simulink model "vehicle_model_paper_2017"  (R2019b)
settings: Solver=ode15s  StartTime=0.0  StopTime=30  RelTol=1e-3  AbsTol=1e-6
values from neighbouring files (symbols this model uses):
  Cr = 0.015    [parameter_values.m]
  Ctr_data = [2.2320 2.0750 1.9750 1.8460 1.7200 1.5640 1.4090 1.2540 1.0960 1.0800 1.0610 1.0430 1.0280 1.0120 1.002 1.002 1.001 0.9980 0.9990 1.001 1.002]    [parameter_values.m]
  DOWN_TABLE = [ ... (first row only)    [parameter_values.m]
  DOWN_TH_BP = [0 2.2352 17.8816 22.352 40.2336 44.704]    [parameter_values.m]
  g = 9.8    [parameter_values.m]
  gear_ratio = [2.34 1.450 1.000 0.68]    [parameter_values.m]
  Iei = 0.224    [parameter_values.m]
  Kb = 20    [parameter_values.m]
  Kc = 1    [parameter_values.m]
  Ktc_data = [ 137.4652 137.0650 135.8644 135.6644 137.5653 140.3666 145.2689 152.8725 162.9773 164.2779 166.1788 167.9797 170.0807 172.7820 175.3832 179.5852 183.5871 189.8901  197.6938 215.9024 244.5160 ]    [parameter_values.m]
  Ktc_ni_ne = [0 0.1000 0.2000 0.3000 0.4000 0.5000 0.6000 0.7000 0.8000 0.8100 0.8200 0.8300 0.8400 0.8500 0.8600 0.8700 0.8800 0.8900 0.9000 0.9200 0.9400]    [parameter_values.m]
  m = 1500.5    [parameter_values.m]
  r = 0.326    [parameter_values.m]
  Rf = 3.28    [parameter_values.m]
  rhoACd = 0.98    [parameter_values.m]
  taub = 0.2    [parameter_values.m]
  Te_data = [ ... (first row only)    [parameter_values.m]
  Te_rpm = [800:400:4800]    [parameter_values.m]
  Te_throtle = [0 20 30 40 50 60 70 80 90 100] / 100    [parameter_values.m]
  UP_TABLE = [ ... (first row only)    [parameter_values.m]
  UP_TH_BP = [ 0 11.176 15.6464 22.352 40.2336 44.704]    [parameter_values.m]
undefined symbols (not defined in the file or in its folder): sigbuilder_block
settings Model: DataTypeOverride=Double  MinMaxOverflowLogging=ForceOff  Creator=ignisgravitas  LastModifiedBy=sls-1
settings SolverCC: MaxOrder=2
settings DebuggingCC: ArithmeticOperatorsInVariantConditions=warning
settings SFSimCC: CustomCodeUndefinedFunction=UseInterfaceOnly

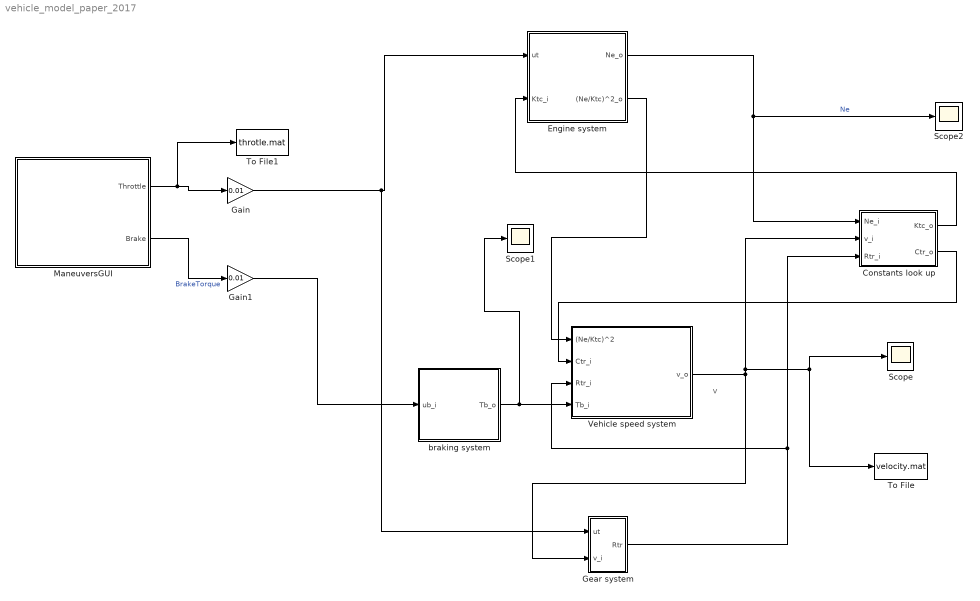
== system vehicle_model_paper_2017 ==
  note: v
  Constants look up : Subsystem
  Engine system : Subsystem
  Gain : Gain  Gain=0.01
  Gain1 : Gain  Gain=0.01
  Gear system : Subsystem
  ManeuversGUI : Subsystem  Tag=STV Subsys  LoadFcn=sigbuilder_block('load');  StartFcn=sigbuilder_block('start');  StopFcn=sigbuilder_block('stop');  ClipboardFcn=sigbuilder_block('clipboard');  mask(Sigbuilder block){tuvar=[0:10]}
      mask help: Sigbuilder GUI
      mask init:
      | tuvar = sigbuilder_block('maskInit');
      settings: CopyFcn=sigbuilder_block('copy');  DeleteFcn=sigbuilder_block('delete');  ModelCloseFcn=sigbuilder_block('modelClose');  PreSaveFcn=sigbuilder_block('preSave');  PauseFcn=sigbuilder_block('pause')  ContinueFcn=sigbuilder_block('continue')  NameChangeFcn=sigbuilder_block('namechange');  OpenFcn=sigbuilder_block('open',[152.337 144.758 981.474 499.453 ]);  CloseFcn=sigbuilder_block('close');
      mask Display: plot(0, 0, 100, 100,[2, 2, 32, 32, 2], [68, 8, 8, 68, 68],[32, 2], [38, 38], [32, 19, 2],[53, 60, 44], [32, 17, 17, 2],[16, 16, 31, 31]);txt = getActiveGroup(gcbh);text(2, 100, txt,'verticalAlignment', 'top');
  Scope : Scope
  Scope1 : Scope
  Scope2 : Scope
  To File : ToFile  Filename=velocity.mat  MatrixName=velocity  SaveFormat=Timeseries
  To File1 : ToFile  Filename=throtle.mat  MatrixName=throtle  SaveFormat=Timeseries
  Vehicle speed system : Subsystem
  braking system : Subsystem
  wires:
  Vehicle speed system/1(v_o) -> To File/1, Scope/1, Constants look up/2(v_i), Gear system/2(v_i)
  Constants look up/2("Ctr_o ") -> Vehicle speed system/2(Ctr_i)
  braking system/1(Tb_o) -> Scope1/1, Vehicle speed system/4(Tb_i)
  Engine system/1(Ne_o) -> Scope2/1, Constants look up/1(Ne_i)  "Ne"
  Engine system/2((Ne/Ktc)^2_o) -> Vehicle speed system/1((Ne/Ktc)^2)
  Gear system/1(Rtr) -> Constants look up/3(Rtr_i), Vehicle speed system/3(Rtr_i)
  ManeuversGUI/1(Throttle) -> To File1/1, Gain/1
  Gain/1 -> Gear system/1(ut), Engine system/1(ut)
  ManeuversGUI/2(Brake) -> Gain1/1  "BrakeTorque"
  Gain1/1 -> braking system/1(ub_i)
  Constants look up/1("Ktc_o ") -> Engine system/2(Ktc_i)

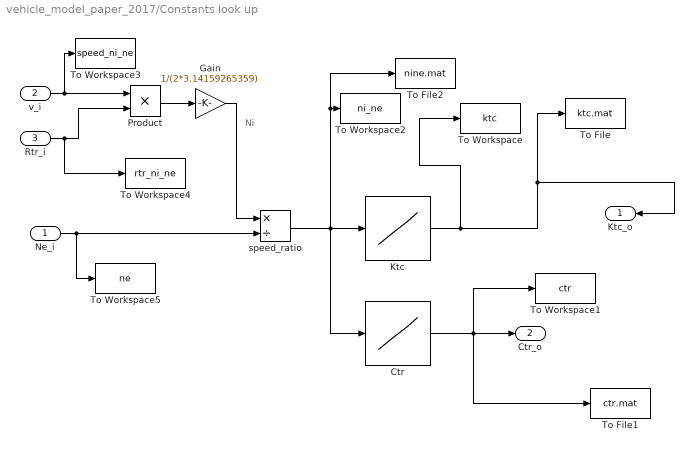
== system vehicle_model_paper_2017/Constants look up ==
  note: Ni
  Ne_i : Inport
  v_i : Inport  Port=2
  Rtr_i : Inport  Port=3
  Ctr : Lookup_n-D  NumberOfTableDimensions=1  BreakpointsForDimension1=Ktc_ni_ne  Table=Ctr_data  ExtrapMethod=Clip  UseLastTableValue=on  InternalRulePriority=Speed  RndMeth=Simplest  InputSameDT=on
  Gain : Gain  Gain=1/(2*3.14159265359)
  "Ktc " : Lookup_n-D  NumberOfTableDimensions=1  BreakpointsForDimension1=Ktc_ni_ne  Table=Ktc_data  ExtrapMethod=Clip  UseLastTableValue=on  InternalRulePriority=Speed  RndMeth=Simplest  InputSameDT=on
  Product : Product
  To File : ToFile  Filename=ktc.mat  SaveFormat=Timeseries
  To File1 : ToFile  Filename=ctr.mat  SaveFormat=Timeseries
  To File2 : ToFile  Filename=nine.mat  SaveFormat=Timeseries
  To Workspace : ToWorkspace  VariableName=ktc  SaveFormat=Timeseries  SampleTime=-1
  To Workspace1 : ToWorkspace  VariableName=ctr  SaveFormat=Timeseries  SampleTime=-1
  To Workspace2 : ToWorkspace  VariableName=ni_ne  SaveFormat=Timeseries  SampleTime=-1
  To Workspace3 : ToWorkspace  VariableName=speed_ni_ne  SaveFormat=Timeseries  SampleTime=-1
  To Workspace4 : ToWorkspace  VariableName=rtr_ni_ne  SaveFormat=Timeseries  SampleTime=-1
  To Workspace5 : ToWorkspace  VariableName=ne  SaveFormat=Timeseries  SampleTime=-1
  speed_ratio : Product  Inputs=*/
  "Ktc_o " : Outport  VectorParamsAs1DForOutWhenUnconnected=off
  "Ctr_o " : Outport  Port=2  VectorParamsAs1DForOutWhenUnconnected=off
  wires:
  Product/1 -> Gain/1
  Gain/1 -> speed_ratio/1
  speed_ratio/1 -> To File2/1, To Workspace2/1, Ctr/1, "Ktc "/1
  "Ktc "/1 -> To Workspace/1, To File/1, "Ktc_o "/1
  v_i/1 -> To Workspace3/1, Product/1
  Ne_i/1 -> To Workspace5/1, speed_ratio/2
  Rtr_i/1 -> To Workspace4/1, Product/2
  Ctr/1 -> To Workspace1/1, To File1/1, "Ctr_o "/1

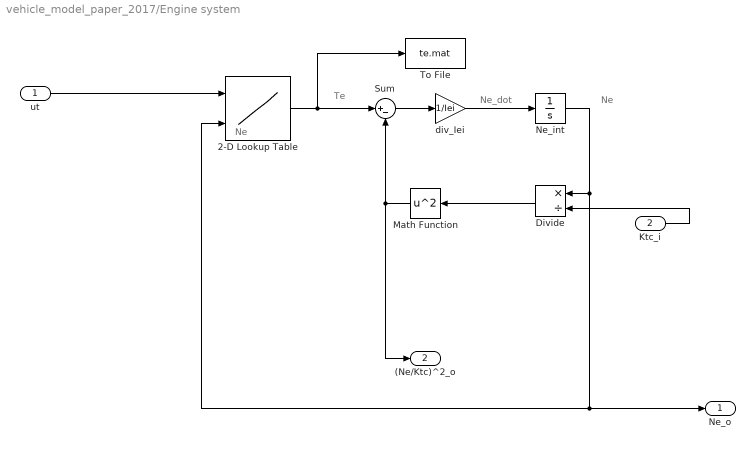
== system vehicle_model_paper_2017/Engine system ==
  note: Ne
  note: Te
  note: Ne_dot
  note: Ne
  ut : Inport
  Ktc_i : Inport  Port=2
  2-D Lookup Table : Lookup_n-D  BreakpointsForDimension1=Te_throtle  BreakpointsForDimension2=Te_rpm  Table=Te_data  UseLastTableValue=on  InternalRulePriority=Speed  InputSameDT=on
  Divide : Product  Inputs=*/
  Math Function : Math  Operator=square  SaturateOnIntegerOverflow=on
  Ne_int : Integrator  InitialCondition=1000
  Sum : Sum  Inputs=|+-
  To File : ToFile  Filename=te.mat  SaveFormat=Timeseries
  div_Iei : Gain  Gain=1/Iei
  Ne_o : Outport  VectorParamsAs1DForOutWhenUnconnected=off
  (Ne/Ktc)^2_o : Outport  Port=2  VectorParamsAs1DForOutWhenUnconnected=off
  wires:
  2-D Lookup Table/1 -> To File/1, Sum/1
  Divide/1 -> Math Function/1
  Sum/1 -> div_Iei/1
  div_Iei/1 -> Ne_int/1
  Math Function/1 -> (Ne/Ktc)^2_o/1, Sum/2
  Ktc_i/1 -> Divide/2
  ut/1 -> 2-D Lookup Table/1
  Ne_int/1 -> 2-D Lookup Table/2, Ne_o/1, Divide/1

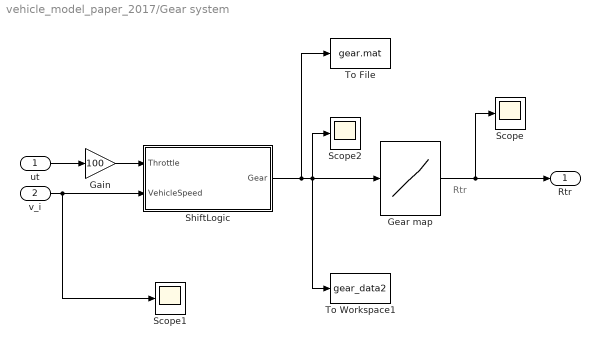
== system vehicle_model_paper_2017/Gear system ==
  note: Rtr
  ut : Inport
  v_i : Inport  Port=2
  Gain : Gain  Gain=100
  Gear map : Lookup_n-D  NumberOfTableDimensions=1  BreakpointsForDimension1=[1 2 3 4]  Table=gear_ratio  OutDataTypeStr=double  SaturateOnIntegerOverflow=on  InputSameDT=on  LockScale=on
  Scope : Scope
  Scope1 : Scope
  Scope2 : Scope
  ShiftLogic : Stateflow chart  TreatAsAtomicUnit=on
  To File : ToFile  Filename=gear.mat  MatrixName=gear  SaveFormat=Timeseries
  To Workspace1 : ToWorkspace  VariableName=gear_data2  SaveFormat=Timeseries  SampleTime=-1
  Rtr : Outport  VectorParamsAs1DForOutWhenUnconnected=off
  wires:
  ShiftLogic/1(Gear) -> To File/1, Scope2/1, To Workspace1/1, Gear map/1
  Gear map/1 -> Scope/1, Rtr/1
  ut/1 -> Gain/1
  Gain/1 -> ShiftLogic/1(Throttle)
  v_i/1 -> ShiftLogic/2(VehicleSpeed), Scope1/1

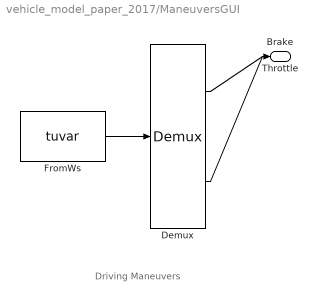
== system vehicle_model_paper_2017/ManeuversGUI ==
  note: Driving Maneuvers
  Demux : Demux  Tag=STV Demux  Outputs=2
  FromWs : FromWorkspace  Tag=STV FromWs  VariableName=tuvar  SampleTime=0
      SigBuilderData=|
      | dataSet(1).timeRange = [0 50]
      | dataSet(1).name = 'Passing Maneuver'
      | dataSet(2).timeRange = [0 50]
      | dataSet(2).name = 'Gradual Acceleration'
      | dataSet(3).timeRange = [0 50]
      | dataSet(3).name = 'Hard braking'
      | dataSet(4).timeRange = [0 50]
      | dataSet(4).name = 'Coasting'
      | sbobj.Groups(1).Name = 'Passing Maneuver'
      | sbobj.Groups(1).Signals(1).Name = 'Throttle'
      | sbobj.Groups(1).Signals(1).XData = [0 14.9 15 50]
      | sbobj.Groups(1).Signals(1).YData = [60 40 100 58.82]
      | sbobj.Groups(1).Signals(2).Name = 'Brake'
      | sbobj.Groups(1).Signals(2).XData = [0 50]
      | sbobj.Groups(1).Signals(2).YData = [0 0]
      | sbobj.Groups(1).TimeRange = [0 50]
      | sbobj.Groups(2).Name = 'Gradual Acceleration'
      | sbobj.Groups(2).Signals(1).Name = 'Throttle'
      | sbobj.Groups(2).Signals(1).XData = [0 15 30 50]
      | sbobj.Groups(2).Signals(1).YData = [0 50 19 100]
      | sbobj.Groups(2).Signals(2).Name = 'Brake'
      | sbobj.Groups(2).Signals(2).XData = [0 50]
      | sbobj.Groups(2).Signals(2).YData = [0 0]
      | sbobj.Groups(2).TimeRange = [0 50]
      | sbobj.Groups(3).Name = 'Hard braking'
      | sbobj.Groups(3).Signals(1).Name = 'Throttle'
      | sbobj.Groups(3).Signals(1).XData = [0 5.1 5.1 50]
      | sbobj.Groups(3).Signals(1).YData = [50 50 1 1]
      | sbobj.Groups(3).Signals(2).Name = 'Brake'
      | sbobj.Groups(3).Signals(2).XData = [0 10 10 50]
      | sbobj.Groups(3).Signals(2).YData = [0 0 20 20]
      | sbobj.Groups(3).TimeRange = [0 50]
      | sbobj.Groups(4).Name = 'Coasting'
      | sbobj.Groups(4).Signals(1).Name = 'Throttle'
      | sbobj.Groups(4).Signals(1).XData = [0 50]
      | sbobj.Groups(4).Signals(1).YData = [30 30]
      | sbobj.Groups(4).Signals(2).Name = 'Brake'
      | sbobj.Groups(4).Signals(2).XData = [0 4 5 7 10 50]
      | sbobj.Groups(4).Signals(2).YData = [0 0 0 0 0 0]
      | sbobj.Groups(4).TimeRange = [0 50]
  Throttle : Outport  Tag=STV Outport  VectorParamsAs1DForOutWhenUnconnected=off
  Brake : Outport  Tag=STV Outport  Port=2  VectorParamsAs1DForOutWhenUnconnected=off
  wires:
  FromWs/1 -> Demux/1
  Demux/1 -> Throttle/1
  Demux/2 -> Brake/1

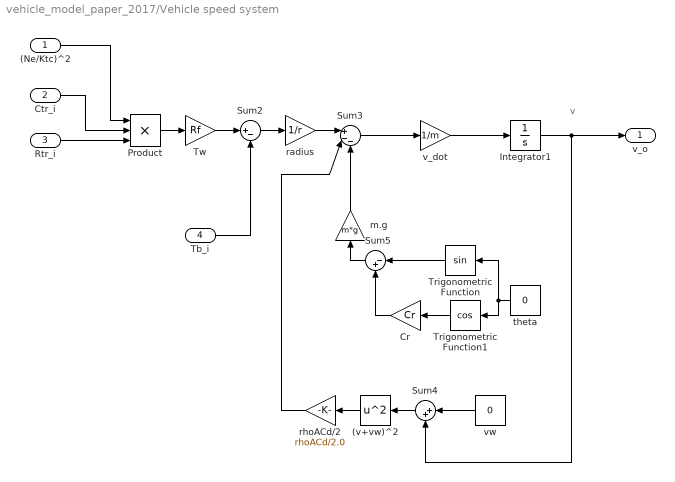
== system vehicle_model_paper_2017/Vehicle speed system ==
  note: v
  (Ne/Ktc)^2 : Inport
  Ctr_i : Inport  Port=2
  Rtr_i : Inport  Port=3
  Tb_i : Inport  Port=4
  " Cr" : Gain  Gain=Cr
  " m.g" : Gain  Gain=m*g
  " rhoACd/2 " : Gain  Gain=rhoACd/2.0
  " v_dot" : Gain  Gain=1/m
  "(v+vw)^2 " : Math  Operator=square  SaturateOnIntegerOverflow=on
  Integrator1 : Integrator  LimitOutput=on  LowerSaturationLimit=0
  Product : Product  Inputs=3
  Sum2 : Sum  Inputs=|+-
  Sum3 : Sum  Inputs=|+--
  Sum4 : Sum  Inputs=|++
  Sum5 : Sum  Inputs=|-+
  Trigonometric Function : Trigonometry
  Trigonometric Function1 : Trigonometry  Operator=cos
  Tw : Gain  Gain=Rf
  "radius " : Gain  Gain=1/r
  theta : Constant  Value=0
  vw : Constant  Value=0
  v_o : Outport  VectorParamsAs1DForOutWhenUnconnected=off
  wires:
  Trigonometric Function1/1 -> " Cr"/1
  Integrator1/1 -> v_o/1, Sum4/2
  Sum4/1 -> "(v+vw)^2 "/1
  " rhoACd/2 "/1 -> Sum3/2
  vw/1 -> Sum4/1
  "(v+vw)^2 "/1 -> " rhoACd/2 "/1
  theta/1 -> Trigonometric Function1/1, Trigonometric Function/1
  Tw/1 -> Sum2/1
  Tb_i/1 -> Sum2/2
  (Ne/Ktc)^2/1 -> Product/1
  Product/1 -> Tw/1
  Rtr_i/1 -> Product/3
  Sum2/1 -> "radius "/1
  " Cr"/1 -> Sum5/2
  Ctr_i/1 -> Product/2
  " v_dot"/1 -> Integrator1/1
  "radius "/1 -> Sum3/1
  Sum3/1 -> " v_dot"/1
  Sum5/1 -> " m.g"/1
  " m.g"/1 -> Sum3/3
  Trigonometric Function/1 -> Sum5/1

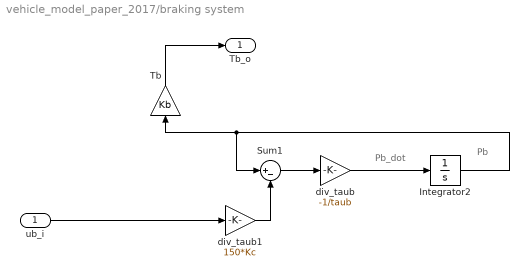
== system vehicle_model_paper_2017/braking system ==
  note: Pb_dot
  note: Pb
  ub_i : Inport
  Integrator2 : Integrator
  Sum1 : Sum  Inputs=|+-
  Tb : Gain  Gain=Kb
  div_taub : Gain  Gain=-1/taub
  div_taub1 : Gain  Gain=150*Kc
  Tb_o : Outport  VectorParamsAs1DForOutWhenUnconnected=off
  wires:
  Sum1/1 -> div_taub/1
  div_taub/1 -> Integrator2/1
  div_taub1/1 -> Sum1/2
  ub_i/1 -> div_taub1/1
  Integrator2/1 -> Tb/1, Sum1/1
  Tb/1 -> Tb_o/1

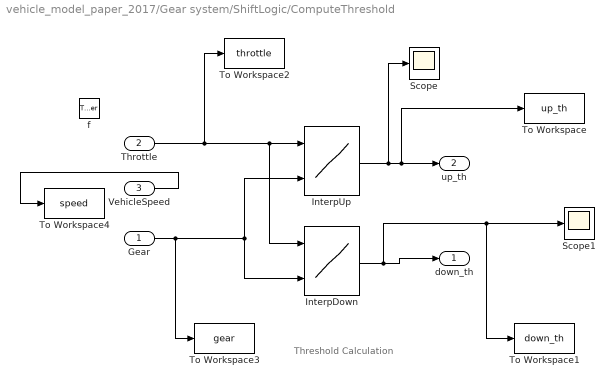
== system vehicle_model_paper_2017/Gear system/ShiftLogic/ComputeThreshold ==
  note: Threshold Calculation
  Gear : Inport
  Throttle : Inport  Port=2
  VehicleSpeed : Inport  Port=3
  f : TriggerPort  TriggerType=function-call  VariantControl=(inherit)
      settings: CopyFcn=Stateflow.SLINSF.SimulinkMan.removeBlockPreDeleteFcn  PreDeleteFcn=Stateflow.SLINSF.SimulinkMan.unsafePredeleteFcn
  InterpDown : Lookup_n-D  BreakpointsForDimension1=DOWN_TH_BP  BreakpointsForDimension2=[1:4]  Table=DOWN_TABLE  ExtrapMethod=Clip  UseLastTableValue=on  OutDataTypeStr=double  LockScale=on
  InterpUp : Lookup_n-D  BreakpointsForDimension1=UP_TH_BP  BreakpointsForDimension2=[1:4]  Table=UP_TABLE  ExtrapMethod=Clip  OutDataTypeStr=double  LockScale=on
  Scope : Scope
  Scope1 : Scope
  To Workspace : ToWorkspace  VariableName=up_th  SaveFormat=Timeseries  SampleTime=-1
  To Workspace1 : ToWorkspace  VariableName=down_th  SaveFormat=Timeseries  SampleTime=-1
  To Workspace2 : ToWorkspace  VariableName=throttle  SaveFormat=Timeseries  SampleTime=-1
  To Workspace3 : ToWorkspace  VariableName=gear  SaveFormat=Timeseries  SampleTime=-1
  To Workspace4 : ToWorkspace  VariableName=speed  SaveFormat=Timeseries  SampleTime=-1
  down_th : Outport  InitialOutput=0  VectorParamsAs1DForOutWhenUnconnected=off
  up_th : Outport  Port=2  InitialOutput=0  VectorParamsAs1DForOutWhenUnconnected=off
  wires:
  InterpDown/1 -> To Workspace1/1, Scope1/1, down_th/1
  Throttle/1 -> To Workspace2/1, InterpDown/1, InterpUp/1
  Gear/1 -> To Workspace3/1, InterpDown/2, InterpUp/2
  InterpUp/1 -> Scope/1, To Workspace/1, up_th/1
  VehicleSpeed/1 -> To Workspace4/1

== stateflow chart vehicle_model_paper_2017/Gear system/ShiftLogic ==
  settings: updateMethod=DISCRETE  sampleTime=0.01
  state gear_state [parallel]
    settings: executionOrder=1
    state first
      entry:
      Gear = 1;
    state second
      entry:
      Gear = 2;
    state third
      entry:
      Gear = 3;
    state fourth
      entry:
      Gear = 4;
    (default) -> first
    second -> third [order 1] : UP
    first -> second : UP
    third -> fourth [order 1] : UP
    third -> second [order 2] : DOWN
    second -> first [order 2] : DOWN
    fourth -> third : DOWN
  state selection_state [parallel]
    during:
    [down_th, up_th] = ComputeThreshold(Gear,Throttle, VehicleSpeed);
    settings: executionOrder=2
    state steady_state
    state upshifting
    state downshifting
    (default) -> steady_state
    steady_state -> upshifting [order 1] : [VehicleSpeed > up_th]
    steady_state -> downshifting [order 2] : [VehicleSpeed < down_th]
    downshifting -> steady_state [order 1] : [VehicleSpeed > down_th]
    downshifting -> steady_state [order 2] : [elapsed('sec') >= 0.08 && VehicleSpeed <= down_th]
        | {gear_state.DOWN}
    upshifting -> steady_state [order 1] : [elapsed('sec') >= 0.08 && VehicleSpeed >= up_th]
        | {gear_state.UP}
    upshifting -> steady_state [order 2] : [VehicleSpeed < up_th]
  state [down_th,up_th] = ComputeThreshold(Gear,Throttle,VehicleSpeed) [function]
  data: Gear function_input; Throttle function_input; down_th function_output; up_th function_output; VehicleSpeed function_input; Throttle input double; VehicleSpeed input double; Gear output fixdt(0,8,5) [1..4]; TWAIT parameter fixdt(0,8,6); down_th local double; up_th local double
  events: DOWN local EITHER_EDGE_EVENT; UP local EITHER_EDGE_EVENT
